simulink model "Aufgabe_4_3_3_Drehtellers2023a"  (R2024a)
settings: Solver=ode3  StartTime=0.0  StopTime=10.0  FixedStep=0.01  RelTol=1e-3
values from neighbouring files (symbols this model uses):
  A = 5    [Aufgabe_4_3_3_Parameter_Drehtellers.m]
  I = 0.5    [Aufgabe_4_3_3_Parameter_Drehtellers.m]
  igetr = 1080    [Aufgabe_4_3_3_Parameter_Drehtellers.m]
  K = 8    [Aufgabe_4_3_3_Parameter_Drehtellers.m]
  MRK = 1    [Aufgabe_4_3_3_Parameter_Drehtellers.m]
  PHI = 0.001    [Aufgabe_4_3_3_Parameter_Drehtellers.m]
  Ra = 40    [Aufgabe_4_3_3_Parameter_Drehtellers.m]
  U = 24    [Aufgabe_4_3_3_Parameter_Drehtellers.m]
settings Model: Creator=ASUS  LastModifiedBy=ASUS

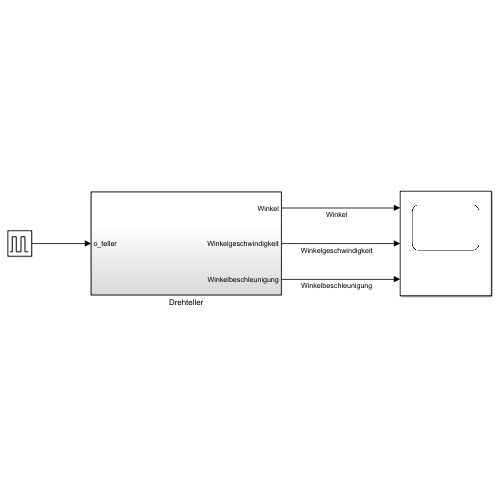
[thumbnail: Simulink's stored preview of the top-level diagram]
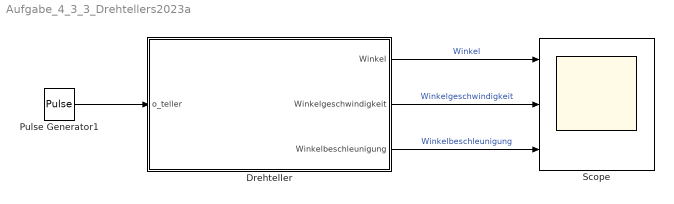
== system Aufgabe_4_3_3_Drehtellers2023a ==
  Drehteller : Subsystem
  Pulse Generator1 : DiscretePulseGenerator  PulseType=Time based  PulseWidth=50
  Scope : Scope  NumInputPorts=3
  wires:
  Pulse Generator1/1 -> Drehteller/1(o_teller)
  Drehteller/1(Winkel) -> Scope/1  "Winkel"
  Drehteller/2(Winkelgeschwindigkeit) -> Scope/2  "Winkelgeschwindigkeit"
  Drehteller/3(Winkelbeschleunigung) -> Scope/3  "Winkelbeschleunigung"

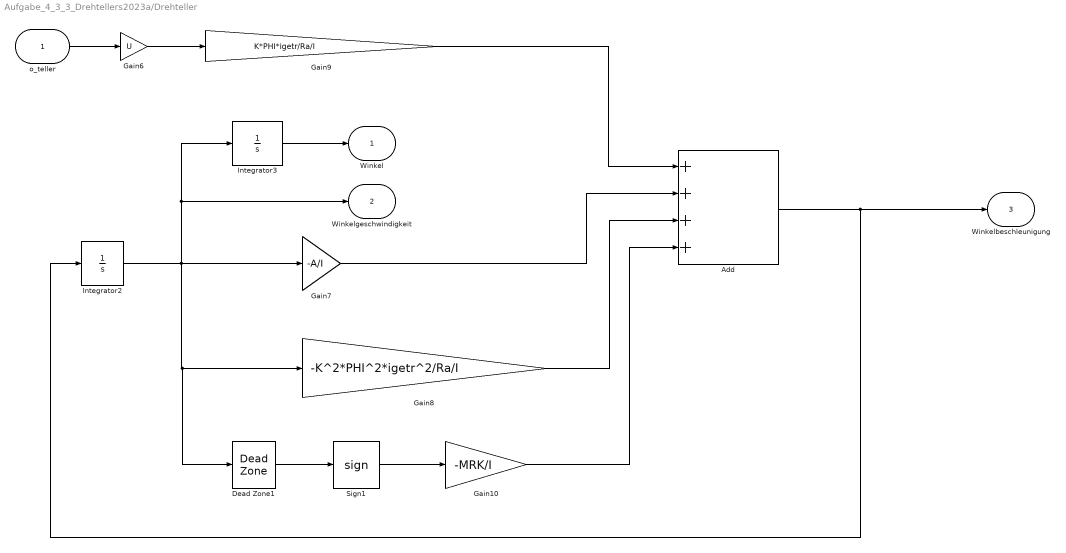
== system Aufgabe_4_3_3_Drehtellers2023a/Drehteller ==
  o_teller : Inport
  Add : Sum  Inputs=++++
  Dead Zone1 : DeadZone
  Gain10 : Gain  Gain=-MRK/I
  Gain6 : Gain  Gain=U
  Gain7 : Gain  Gain=-A/I
  Gain8 : Gain  Gain=-K^2*PHI^2*igetr^2/Ra/I
  Gain9 : Gain  Gain=K*PHI*igetr/Ra/I
  Integrator2 : Integrator
  Integrator3 : Integrator
  Sign1 : Signum
  Winkel : Outport
  Winkelgeschwindigkeit : Outport  Port=2
  Winkelbeschleunigung : Outport  Port=3
  wires:
  Gain6/1 -> Gain9/1
  Sign1/1 -> Gain10/1
  Gain7/1 -> Add/2
  Gain10/1 -> Add/4
  Gain8/1 -> Add/3
  Integrator3/1 -> Winkel/1
  Integrator2/1 -> Winkelgeschwindigkeit/1, Integrator3/1, Dead Zone1/1, Gain8/1, Gain7/1
  Gain9/1 -> Add/1
  Dead Zone1/1 -> Sign1/1
  o_teller/1 -> Gain6/1
  Add/1 -> Integrator2/1, Winkelbeschleunigung/1
